simulink model "PNEUMA"  (R2023b)
settings: Solver=ode23tb  StartTime=0  StopTime=3600  FixedStep=0.001  MaxStep=time_step_new  RelTol=0.01  EnableMultiTasking=on
values from neighbouring files (symbols this model uses):
  A = 20.9    [Gas_Exchange_IC.m]    (also in getPneumonia.m = (LF1-LF2)/(1-exp(Rresolve*(t2(end)-t2(1)))))
  a1 = 0.3836    [Dissociation_Spencer_IC.m]    (also in Gas_Exchange_IC.m; Respiratory_IC.m)
  a2 = 1.819    [Dissociation_Spencer_IC.m]    (also in Gas_Exchange_IC.m; Respiratory_IC.m)
  alpha1 = 0.02598    [Dissociation_Spencer_IC.m]    (also in Gas_Exchange_IC.m; Respiratory_IC.m)
  alpha2 = 0.05591    [Dissociation_Spencer_IC.m]    (also in Gas_Exchange_IC.m; Respiratory_IC.m)
  B = 92.8    [Gas_Exchange_IC.m]    (also in getPneumonia.m = LungFunction(end)-A)
  beta1 = 0.012275    [Dissociation_Spencer_IC.m]    (also in Gas_Exchange_IC.m; Respiratory_IC.m)
  beta2 = 0.03255    [Dissociation_Spencer_IC.m]    (also in Gas_Exchange_IC.m; Respiratory_IC.m)
  C = 10570    [Gas_Exchange_IC.m]
  C1 = 9    [Dissociation_Spencer_IC.m]    (also in Gas_Exchange_IC.m; Respiratory_IC.m)
  C2 = 87.00    (= 87)    [Dissociation_Spencer_IC.m]    (also in Gas_Exchange_IC.m; Respiratory_IC.m)
  Circadian_Period = 24    [Respiratory_IC.m]    (also in State_UA_Khoo_IC.m)
  CvCO2IC = 0.5116    [Body_Khoo_IC.m]    (also in Gas_Exchange_IC.m; Respiratory_IC.m = 0.5247)
  CvO2IC = 0.1672    [Body_Khoo_IC.m]    (also in Gas_Exchange_IC.m; Respiratory_IC.m = 0.1639)
  D = -5.251    [Gas_Exchange_IC.m]
  Dead1CO2IC = 0.1020    (= 0.102)    [Dead_Space_Khoo_IC.m]    (also in Gas_Exchange_IC.m; Respiratory_IC.m = 39.5616)
  Dead1O2IC = 149.8824    [Dead_Space_Khoo_IC.m]    (also in Gas_Exchange_IC.m; Respiratory_IC.m = 104.3637)
  Dead2CO2IC = 0.5274    [Dead_Space_Khoo_IC.m]    (also in Gas_Exchange_IC.m; Respiratory_IC.m = 39.6736)
  Dead2O2IC = 149.3923    [Dead_Space_Khoo_IC.m]    (also in Gas_Exchange_IC.m; Respiratory_IC.m = 104.2258)
  Dead3CO2IC = 2.2996    [Dead_Space_Khoo_IC.m]    (also in Gas_Exchange_IC.m; Respiratory_IC.m = 39.8127)
  Dead3O2IC = 147.3503    [Dead_Space_Khoo_IC.m]    (also in Gas_Exchange_IC.m; Respiratory_IC.m = 104.0505)
  Dead4CO2IC = 8.2293    [Dead_Space_Khoo_IC.m]    (also in Gas_Exchange_IC.m; Respiratory_IC.m = 40.0061)
  Dead4O2IC = 140.5179    [Dead_Space_Khoo_IC.m]    (also in Gas_Exchange_IC.m; Respiratory_IC.m = 103.8005)
  Dead5CO2IC = 22.0757    [Dead_Space_Khoo_IC.m]    (also in Gas_Exchange_IC.m; Respiratory_IC.m = 40.3359)
  Dead5O2IC = 124.5641    [Dead_Space_Khoo_IC.m]    (also in Gas_Exchange_IC.m; Respiratory_IC.m = 103.3579)
  DtotalIC = 0.3    [NeuroMuscular_IC.m]    (also in Respiratory_IC.m = 0.32)
  E_CW = 5    [Pleural_Schuessler_IC.m]    (also in Pmus_Flow_Younes_IC.m; Resp_Mech_IC.m; Respiratory_IC.m)
  E_L = 5    [Pleural_Schuessler_IC.m]    (also in Pmus_Flow_Younes_IC.m; Resp_Mech_IC.m; Respiratory_IC.m)
  fc = 0.4/60    (= 0.00666666666667)    [Respiratory_IC.m]    (also in State_UA_Khoo_IC.m)
  fcs_max = 47.78    [Cardiovascular_IC.m]    (also in Reflex_Ursino_IC.m)
  fcs_min = 2.52    [Cardiovascular_IC.m]    (also in Reflex_Ursino_IC.m)
  fcs_zero = 25    [Respiratory_IC.m]
  FlowIC = 0    [Pmus_Flow_Younes_IC.m]    (also in Resp_Mech_IC.m; Respiratory_IC.m)
  fp_inf = 6.3    [Respiratory_IC.m]
  fp_zero = 3.2    [Respiratory_IC.m]
  fs_inf = 2.10    (= 2.1)    [Respiratory_IC.m]
  fs_zero = 16.11    [Respiratory_IC.m]
  ftbs_min = 0.1    [Cardiovascular_IC.m]    (also in SA_Node_Ursino_IC.m)
  gc = 0.008/60    (= 0.000133333333333)    [Respiratory_IC.m]    (also in State_UA_Khoo_IC.m)
  h = 0.0183    [Brain_Khoo_IC.m]    (also in Gas_Exchange_IC.m; Respiratory_IC.m)
  HP_basal = 0.58    [Cardiovascular_IC.m]    (also in SA_Node_Ursino_IC.m)
  Ic = 45    [Gas_Exchange_IC.m]    (also in Respiratory_IC.m; Vent_Drive_Khoo_IC.m)
  IpCO2 = 38    [Gas_Exchange_IC.m]    (also in Respiratory_IC.m; Vent_Drive_Khoo_IC.m)
  IpO2 = 102.4    [Gas_Exchange_IC.m]    (also in Respiratory_IC.m; Vent_Drive_Khoo_IC.m)
  K1 = 13    [Dissociation_Spencer_IC.m]    (also in Gas_Exchange_IC.m; Respiratory_IC.m)
  K2 = 194.4    [Dissociation_Spencer_IC.m]    (also in Gas_Exchange_IC.m; Respiratory_IC.m)
  k_cs = 11.758    [Cardiovascular_IC.m]    (also in Reflex_Ursino_IC.m)
  k_p = 7.06    [Respiratory_IC.m]
  k_s = 0.07    [Respiratory_IC.m]
  lambda = 863    [Gas_Exchange_IC.m]    (also in Lungs_Khoo_IC.m; Respiratory_IC.m)
  Mech_Vent_pressure = 17    [Mech_vent_test.m]
  MRbCO2 = 0.0517    [Brain_Khoo_IC.m]    (also in Gas_Exchange_IC.m; Respiratory_IC.m)
  MRCO2 = 0.0033    [Body_Khoo_IC.m]    (also in Gas_Exchange_IC.m; Respiratory_IC.m)
  MRO2 = 0.0038    [Body_Khoo_IC.m]    (also in Gas_Exchange_IC.m; Respiratory_IC.m)
  NM_block_gain = 1    [Mech_vent_test.m]
  PACO2_delayIC = 39.6041    [Cardio_Mix_Lange_IC.m]    (also in Gas_Exchange_IC.m; Respiratory_IC.m = 40.4448)
  PaCO2firstIC = 0.2150    (= 0.215)    [Cardio_Mix_Lange_IC.m]    (also in Gas_Exchange_IC.m; Respiratory_IC.m = -0.2465)
  PACO2IC = 37.1484    [Gas_Exchange_IC.m]    (also in Lungs_Khoo_IC.m; Respiratory_IC.m = 40.9432)
  PaCO2secondIC = 38.4577    [Cardio_Mix_Lange_IC.m]    (also in Gas_Exchange_IC.m; Respiratory_IC.m = 40.3928)
  PAO2_delayIC = 103.8436    [Cardio_Mix_Lange_IC.m]    (also in Gas_Exchange_IC.m; Respiratory_IC.m = 103.1223)
  PaO2firstIC = -0.2838    [Cardio_Mix_Lange_IC.m]    (also in Gas_Exchange_IC.m; Respiratory_IC.m = 0.3557)
  PAO2IC = 107.1983    [Gas_Exchange_IC.m]    (also in Lungs_Khoo_IC.m; Respiratory_IC.m = 102.5153)
  PaO2secondIC = 105.4828    [Cardio_Mix_Lange_IC.m]    (also in Gas_Exchange_IC.m; Respiratory_IC.m = 103.1435)
  PbCO2IC = 48.2858    [Brain_Khoo_IC.m]    (also in Gas_Exchange_IC.m; Respiratory_IC.m = 48.5383)
  PICO2 = 0    [Dead_Space_Khoo_IC.m]    (also in Gas_Exchange_IC.m; Respiratory_IC.m)
  PIO2 = 150    [Dead_Space_Khoo_IC.m]    (also in Gas_Exchange_IC.m; Respiratory_IC.m)
  PIO2_change = -90    [Mech_vent_test.m]    (also in Respiratory_IC.m = 0)
  Pn = 90    [Cardiovascular_IC.m]    (also in Reflex_Ursino_IC.m)
  Pt_frcIC1 = 0    [Pmus_Flow_Younes_IC.m]    (also in Resp_Mech_IC.m; Respiratory_IC.m)
  Pt_frcIC2 = 0    [Pmus_Flow_Younes_IC.m]    (also in Resp_Mech_IC.m; Respiratory_IC.m)
  QdBo = 0.8333    [Brain_Khoo_IC.m]    (also in Gas_Exchange_IC.m; Respiratory_IC.m)
  R_AW = 1.27    [Pleural_Schuessler_IC.m]    (also in Pmus_Flow_Younes_IC.m; Resp_Mech_IC.m; Respiratory_IC.m)
  R_CW = 1.03    [Pleural_Schuessler_IC.m]    (also in Pmus_Flow_Younes_IC.m; Resp_Mech_IC.m; Respiratory_IC.m)
  R_L = 1.69    [Pleural_Schuessler_IC.m]    (also in Pmus_Flow_Younes_IC.m; Resp_Mech_IC.m; Respiratory_IC.m)
  RC = 0.06    [Pleural_Schuessler_IC.m]    (also in Pmus_Flow_Younes_IC.m; Resp_Mech_IC.m; Respiratory_IC.m)
  rc = 0.2/60    (= 0.00333333333333)    [Respiratory_IC.m]    (also in State_UA_Khoo_IC.m)
  SbCO2 = 0.3600    (= 0.36)    [Brain_Khoo_IC.m]    (also in Gas_Exchange_IC.m; Respiratory_IC.m)
  SCO2 = 0.0043    [Brain_Khoo_IC.m]    (also in Gas_Exchange_IC.m; Respiratory_IC.m)
  SWAo = 0.007    [Respiratory_IC.m]    (also in State_UA_Khoo_IC.m)
  T1 = 1    [Cardio_Mix_Lange_IC.m]    (also in Gas_Exchange_IC.m; Respiratory_IC.m)
  T2 = 2    [Cardio_Mix_Lange_IC.m]    (also in Gas_Exchange_IC.m; Respiratory_IC.m)
  t_end_new = 4*24*60*60    (= 345600)    [Mech_vent_test.m]
  t_end_UA = 0    [Respiratory_IC.m]    (also in State_UA_Khoo_IC.m)
  t_Mech_Vent_duration = 0    [Mech_vent_test.m]
  t_Mech_Vent_start = 0    [Mech_vent_test.m]
  t_Mueller_duration = 0    [NeuroMuscular_IC.m]
  t_Mueller_insp = 0    [NeuroMuscular_IC.m]
  t_Mueller_start = 0    [NeuroMuscular_IC.m]
  t_NM_block_duration = 0    [Mech_vent_test.m]
  t_NM_block_start = 0    [Mech_vent_test.m]
  t_O2_duration = 0    [Mech_vent_test.m]    (also in Respiratory_IC.m)
  t_O2_start = 0    [Mech_vent_test.m]    (also in Respiratory_IC.m)
  t_start_new = 0    [Mech_vent_test.m]
  t_start_UA = 0    [Respiratory_IC.m]    (also in State_UA_Khoo_IC.m)
  t_valsalva_duration = 0    [NeuroMuscular_IC.m]
  t_valsalva_insp = 0    [NeuroMuscular_IC.m]
  t_valsalva_start = 0    [NeuroMuscular_IC.m]
  time_step = time_step    [acquire_data.m]    (also in acquire_data_save.m)
  VC = 5    [Pmus_Flow_Younes_IC.m]    (also in Resp_Mech_IC.m; Respiratory_IC.m)
  Vdead1 = 0.03    [Dead_Space_Khoo_IC.m]    (also in Gas_Exchange_IC.m; Respiratory_IC.m)
  Vdead2 = 0.03    [Dead_Space_Khoo_IC.m]    (also in Gas_Exchange_IC.m; Respiratory_IC.m)
  Vdead3 = 0.03    [Dead_Space_Khoo_IC.m]    (also in Gas_Exchange_IC.m; Respiratory_IC.m)
  Vdead4 = 0.03    [Dead_Space_Khoo_IC.m]    (also in Gas_Exchange_IC.m; Respiratory_IC.m)
  Vdead5 = 0.03    [Dead_Space_Khoo_IC.m]    (also in Gas_Exchange_IC.m; Respiratory_IC.m)
  Ventilator_rate = 12    [Mech_vent_test.m]
  VTCO2 = 15    [Body_Khoo_IC.m]    (also in Gas_Exchange_IC.m; Respiratory_IC.m)
  VtIC = 0    [Pmus_Flow_Younes_IC.m]    (also in Resp_Mech_IC.m; Respiratory_IC.m)
  VTO2 = 6    [Body_Khoo_IC.m]    (also in Gas_Exchange_IC.m; Respiratory_IC.m)
  Z = 0.0227    [Dissociation_Spencer_IC.m]    (also in Gas_Exchange_IC.m; Respiratory_IC.m)
undefined symbols (not defined in the file or in its folder): A_0_ua, alpha_E_FFA_Heart, alpha_E_FFA_muscle, alpha_E_GLC_Heart, alpha_E_GLC_muscle, alpha_E_GLY_muscle, alpha_E_PYR_muscle, alpha_E_TGL_adipose, alpha_E_TGL_GI, alpha_E_TGL_Heart, alpha_E_TGL_muscle, Arousal_UAIC, C_ua_awake, Cbp, Cbv, Ce_0, Cep, Cev, Chp, Chv, Cla, Clamp_class, Cmp, Cmv, Cpa, CPAP_pressure, Cpp, Cpv, Cra, Csa, Csp, Csv, CvbO2_n, CvhO2_n, CvmO2_n, DAY, delay, DietBlock, Dx, Fb, fchemo_max, fchemo_min, fchemoIC, flsIC, Ftas_I0, ftas_min, ftas_r0, FVC_activation, gain_E, Gamma, Gas_sleep, Gas_sleepM, Gb, Gblock, GbO2, Gbs_sleep, gcc_sa, gcc_sb, gcc_sp, Gclamp ... (+144)
libraries: simulink x4, dspstat3 x4, simulink_extras x2
(part 5 of 8)

== system PNEUMA/Display Panels/Saving CARDIORESPIRATORY/If Action Subsystem ==
  In1 : Inport
  Action Port : ActionPort  ActionPortLabel=if((u1>777600)&(u1<=864000))
  "SI/HR/ABP To File " : ToFile  Filename=CARDIORESPIRATORYday10.mat  MatrixName=CARDIORESPIRATORY
  wires:
  In1/1 -> "SI/HR/ABP To File "/1

== system PNEUMA/Display Panels/Saving CARDIORESPIRATORY/Switch Case Action Subsystem ==
  In1 : Inport
  Action Port : ActionPort  ActionPortLabel=case [ 0 ]:
  To File : ToFile  Filename=CARDIORESPIRATORY1.mat  MatrixName=CARDIORESPIRATORY  SampleTime=sampletime
  wires:
  In1/1 -> To File/1

== system PNEUMA/Display Panels/Saving CARDIORESPIRATORY/Switch Case Action Subsystem1 ==
  In1 : Inport
  Action Port : ActionPort  ActionPortLabel=case [ 1 ]:
  To File : ToFile  Filename=CARDIORESPIRATORY2.mat  MatrixName=CARDIORESPIRATORY  SampleTime=sampletime
  wires:
  In1/1 -> To File/1

== system PNEUMA/Display Panels/Saving CARDIORESPIRATORY/Switch Case Action Subsystem2 ==
  In1 : Inport
  Action Port : ActionPort  ActionPortLabel=case [ 2 ]:
  To File : ToFile  Filename=CARDIORESPIRATORY3.mat  MatrixName=CARDIORESPIRATORY  SampleTime=sampletime
  wires:
  In1/1 -> To File/1

== system PNEUMA/Display Panels/Saving CARDIORESPIRATORY/Switch Case Action Subsystem3 ==
  In1 : Inport
  Action Port : ActionPort  ActionPortLabel=default:
  To File : ToFile  Filename=CARDIORESPIRATORY10.mat  MatrixName=CARDIORESPIRATORY  SampleTime=sampletime
  wires:
  In1/1 -> To File/1

== system PNEUMA/Display Panels/Saving CARDIORESPIRATORY/Switch Case Action Subsystem4 ==
  In1 : Inport
  Action Port : ActionPort  ActionPortLabel=case [ 3 ]:
  To File : ToFile  Filename=CARDIORESPIRATORY4.mat  MatrixName=CARDIORESPIRATORY  SampleTime=sampletime
  wires:
  In1/1 -> To File/1

== system PNEUMA/Display Panels/Saving CARDIORESPIRATORY/Switch Case Action Subsystem5 ==
  In1 : Inport
  Action Port : ActionPort  ActionPortLabel=case [ 4 ]:
  To File : ToFile  Filename=CARDIORESPIRATORY5.mat  MatrixName=CARDIORESPIRATORY  SampleTime=sampletime
  wires:
  In1/1 -> To File/1

== system PNEUMA/Display Panels/Saving CARDIORESPIRATORY/Switch Case Action Subsystem6 ==
  In1 : Inport
  Action Port : ActionPort  ActionPortLabel=case [ 5 ]:
  To File : ToFile  Filename=CARDIORESPIRATORY6.mat  MatrixName=CARDIORESPIRATORY  SampleTime=sampletime
  wires:
  In1/1 -> To File/1

== system PNEUMA/Display Panels/Saving CARDIORESPIRATORY/Switch Case Action Subsystem7 ==
  In1 : Inport
  Action Port : ActionPort  ActionPortLabel=case [ 6 ]:
  To File : ToFile  Filename=CARDIORESPIRATORY7.mat  MatrixName=CARDIORESPIRATORY  SampleTime=sampletime
  wires:
  In1/1 -> To File/1

== system PNEUMA/Display Panels/Saving CARDIORESPIRATORY/Switch Case Action Subsystem8 ==
  In1 : Inport
  Action Port : ActionPort  ActionPortLabel=case [ 7 ]:
  To File : ToFile  Filename=CARDIORESPIRATORY8.mat  MatrixName=CARDIORESPIRATORY  SampleTime=sampletime
  wires:
  In1/1 -> To File/1

== system PNEUMA/Display Panels/Saving CARDIORESPIRATORY/Switch Case Action Subsystem9 ==
  In1 : Inport
  Action Port : ActionPort  ActionPortLabel=case [ 8 ]:
  To File : ToFile  Filename=CARDIORESPIRATORY9.mat  MatrixName=CARDIORESPIRATORY  SampleTime=sampletime
  wires:
  In1/1 -> To File/1

== system PNEUMA/Display Panels/Saving CARDIO/Switch Case Action Subsystem ==
  In1 : Inport
  Action Port : ActionPort  ActionPortLabel=case [ 0 ]:
  To File : ToFile  Filename=CARDIO1.mat  MatrixName=CARDIO  SampleTime=sampletime
  wires:
  In1/1 -> To File/1

== system PNEUMA/Display Panels/Saving CARDIO/Switch Case Action Subsystem1 ==
  In1 : Inport
  Action Port : ActionPort  ActionPortLabel=case [ 1 ]:
  To File : ToFile  Filename=CARDIO2.mat  MatrixName=CARDIO  SampleTime=sampletime
  wires:
  In1/1 -> To File/1

== system PNEUMA/Display Panels/Saving CARDIO/Switch Case Action Subsystem2 ==
  In1 : Inport
  Action Port : ActionPort  ActionPortLabel=case [ 2 ]:
  To File : ToFile  Filename=CARDIO3.mat  MatrixName=CARDIO  SampleTime=sampletime
  wires:
  In1/1 -> To File/1

== system PNEUMA/Display Panels/Saving CARDIO/Switch Case Action Subsystem3 ==
  In1 : Inport
  Action Port : ActionPort  ActionPortLabel=default:
  To File : ToFile  Filename=CARDIO10.mat  MatrixName=CARDIO  SampleTime=sampletime
  wires:
  In1/1 -> To File/1

== system PNEUMA/Display Panels/Saving CARDIO/Switch Case Action Subsystem4 ==
  In1 : Inport
  Action Port : ActionPort  ActionPortLabel=case [ 3 ]:
  To File : ToFile  Filename=CARDIO4.mat  MatrixName=CARDIO  SampleTime=sampletime
  wires:
  In1/1 -> To File/1

== system PNEUMA/Display Panels/Saving CARDIO/Switch Case Action Subsystem5 ==
  In1 : Inport
  Action Port : ActionPort  ActionPortLabel=case [ 4 ]:
  To File : ToFile  Filename=CARDIO5.mat  MatrixName=CARDIO  SampleTime=sampletime
  wires:
  In1/1 -> To File/1

== system PNEUMA/Display Panels/Saving CARDIO/Switch Case Action Subsystem6 ==
  In1 : Inport
  Action Port : ActionPort  ActionPortLabel=case [ 5 ]:
  To File : ToFile  Filename=CARDIO6.mat  MatrixName=CARDIO  SampleTime=sampletime
  wires:
  In1/1 -> To File/1

== system PNEUMA/Display Panels/Saving CARDIO/Switch Case Action Subsystem7 ==
  In1 : Inport
  Action Port : ActionPort  ActionPortLabel=case [ 6 ]:
  To File : ToFile  Filename=CARDIO7.mat  MatrixName=CARDIO  SampleTime=sampletime
  wires:
  In1/1 -> To File/1

== system PNEUMA/Display Panels/Saving CARDIO/Switch Case Action Subsystem8 ==
  In1 : Inport
  Action Port : ActionPort  ActionPortLabel=case [ 7 ]:
  To File : ToFile  Filename=CARDIO8.mat  MatrixName=CARDIO  SampleTime=sampletime
  wires:
  In1/1 -> To File/1

== system PNEUMA/Display Panels/Saving CARDIO/Switch Case Action Subsystem9 ==
  In1 : Inport
  Action Port : ActionPort  ActionPortLabel=case [ 8 ]:
  To File : ToFile  Filename=CARDIO9.mat  MatrixName=CARDIO  SampleTime=sampletime
  wires:
  In1/1 -> To File/1

== system PNEUMA/Metabolic Control/Display & Storage/Saving G_I_FFA ==
  In1 : Inport
  Clock : Clock
  Gain = 7day : Gain  Gain=1/(3600*24*DAY)
  Rounding Function : Rounding
  Switch Case : SwitchCase  CaseConditions={0,1,2,3,4,5,6,7,8}  SampleTime=sampletime*6
  Switch Case Action Subsystem : Subsystem  TreatAsAtomicUnit=on
  Switch Case Action Subsystem1 : Subsystem  TreatAsAtomicUnit=on
  Switch Case Action Subsystem2 : Subsystem  TreatAsAtomicUnit=on
  Switch Case Action Subsystem3 : Subsystem  TreatAsAtomicUnit=on
  Switch Case Action Subsystem4 : Subsystem  TreatAsAtomicUnit=on
  Switch Case Action Subsystem5 : Subsystem  TreatAsAtomicUnit=on
  Switch Case Action Subsystem6 : Subsystem  TreatAsAtomicUnit=on
  Switch Case Action Subsystem7 : Subsystem  TreatAsAtomicUnit=on
  Switch Case Action Subsystem8 : Subsystem  TreatAsAtomicUnit=on
  Switch Case Action Subsystem9 : Subsystem  TreatAsAtomicUnit=on
  wires:
  Clock/1 -> Gain = 7day/1
  Switch Case/1 -> Switch Case Action Subsystem/Action
  Switch Case/2 -> Switch Case Action Subsystem1/Action
  Switch Case/3 -> Switch Case Action Subsystem2/Action
  Switch Case/10 -> Switch Case Action Subsystem3/Action
  Rounding Function/1 -> Switch Case/1
  In1/1 -> Switch Case Action Subsystem/1(In1), Switch Case Action Subsystem1/1(In1), Switch Case Action Subsystem2/1(In1), Switch Case Action Subsystem4/1(In1), Switch Case Action Subsystem5/1(In1), Switch Case Action Subsystem3/1(In1), Switch Case Action Subsystem9/1(In1), Switch Case Action Subsystem8/1(In1), Switch Case Action Subsystem7/1(In1), Switch Case Action Subsystem6/1(In1)
  Gain = 7day/1 -> Rounding Function/1
  Switch Case/4 -> Switch Case Action Subsystem4/Action
  Switch Case/5 -> Switch Case Action Subsystem5/Action
  Switch Case/6 -> Switch Case Action Subsystem6/Action
  Switch Case/7 -> Switch Case Action Subsystem7/Action
  Switch Case/8 -> Switch Case Action Subsystem8/Action
  Switch Case/9 -> Switch Case Action Subsystem9/Action

== system PNEUMA/Metabolic Control/Epinephrine Regulation on Heart and Muscle/Epi Dynamics ==
  Ftas_r : Inport
  SI : Inport  Port=2
  REM : Inport  Port=3
  Constant1 : Constant  Value=Ce_0
  Ftas_Ce0 : Fcn  Expr=(u(1) - ftas_r0*(1-u(2)*Gas_sleepM)+1)*1e-6
  Ftas_Ce0*(1-SI) : Fcn  Expr=((u(1)>=u(4))*(u(1)-u(4)+0) + (u(1)<u(4))*0)*(1-u(2))*1e-6
  Ftas_Ce0*(1-SI*Gas_SleepM) : Fcn  Expr=((u(1)>=u(4))*(u(1)-u(4)+1) + (u(1)<u(4))*1)*(1-u(2)*Gas_sleepM)*1e-6
  Ftas_REM_Sleeo ABS Fcn REM factor = 0.4 Ftas,r0_metabolic Gas factor_M : Fcn  Expr=(abs(u(1) - ftas_r0*(1-u(2)*Gas_sleepM)+1))^(u(2)*Gas_sleepM)*(1+0.4*u(3))*(1-u(2)*0.6)
  Ftas_REM_Sleep Fcn REM factor = 0.4 Ftas,r0_metabolic Gas factor_M Neg Power : Fcn  Expr=((u(1)>=u(4))*(u(1)-u(4)+1) + (u(1)<u(4))*1)^(-u(2)*Gas_sleepM)*(1+0.4*u(3))*(1-u(2)*0.6)
  Ftas_metabolic : Fcn  Expr=u(1)*(1-u(2)*Gas_sleepM)
  Ftas_r0_metabolic : Fcn  Expr=ftas_r0*(1-u(2)*Gas_sleepM)
  Gain : Gain  Gain=1/tao_e
  Gain1 : Gain  Gain=9
  Integrator : Integrator  InitialCondition=Ce_0
  Mux : Mux  Inputs=2
  Mux1 : Mux
  Product : Product  RndMeth=Zero
  Saturation : Saturate  UpperLimit=3  LowerLimit=0.1
  Sum1 : Sum  Inputs=-++  InputSameDT=on  SaturateOnIntegerOverflow=on  OutDataTypeStr=Inherit: Same as first input
  Terminator : Terminator
  Terminator1 : Terminator
  Terminator2 : Terminator
  Ce(t) : Outport
  W_alphaSYMP : Outport  Port=2
  wires:
  Sum1/1 -> Gain/1
  Integrator/1 -> Sum1/1, Ce(t)/1
  Gain/1 -> Integrator/1
  Constant1/1 -> Product/2
  Product/1 -> Sum1/2
  Mux/1 -> Ftas_r0_metabolic/1, Ftas_metabolic/1
  Ftas_r/1 -> Mux/1
  SI/1 -> Mux/2, Mux1/2
  Ftas_metabolic/1 -> Mux1/1
  REM/1 -> Mux1/3
  Mux1/1 -> Ftas_REM_Sleep Fcn REM factor = 0.4 Ftas,r0_metabolic Gas factor_M Neg Power/1, Ftas_REM_Sleeo ABS Fcn REM factor = 0.4 Ftas,r0_metabolic Gas factor_M/1, Ftas_Ce0*(1-SI)/1, Ftas_Ce0*(1-SI*Gas_SleepM)/1, Ftas_Ce0/1
  Ftas_Ce0/1 -> Terminator1/1
  Ftas_r0_metabolic/1 -> Mux1/4
  Ftas_REM_Sleeo ABS Fcn REM factor = 0.4 Ftas,r0_metabolic Gas factor_M/1 -> Terminator/1
  Ftas_REM_Sleep Fcn REM factor = 0.4 Ftas,r0_metabolic Gas factor_M Neg Power/1 -> Saturation/1
  Saturation/1 -> Product/1, W_alphaSYMP/1
  Gain1/1 -> Sum1/3
  Ftas_Ce0*(1-SI*Gas_SleepM)/1 -> Terminator2/1
  Ftas_Ce0*(1-SI)/1 -> Gain1/1

== system PNEUMA/Metabolic Control/Epinephrine Regulation on Heart and Muscle/Epi Modulation ==
  Ce(t) : Inport
  GI : Subsystem
  GI1 : Subsystem
  Heart : Subsystem
  Heart Fluxes : Scope
  Muscle : Subsystem
  Muscle Fluxes : Scope
  Epi on Heart : Outport
  Epi on Muscle : Outport  Port=2
  Epi on GI : Outport  Port=3
  Epi on adipose : Outport  Port=4
  4Fluxes of Epi in Heart : Outport  Port=5
  5Fluxes of Epi in Muscle : Outport  Port=6
  wires:
  Heart/2(Epi on Heart (Sum)) -> Epi on Heart/1
  Ce(t)/1 -> Heart/1(Ce(t)), Muscle/1(Ce(t)), GI/1(Ce(t)), GI1/1(Ce(t))
  Heart/1(Epi on Heart (Fluxes)) -> Heart Fluxes/1, 4Fluxes of Epi in Heart/1
  Muscle/2(Epi on Muscle(Sum)) -> Epi on Muscle/1
  Muscle/1(Epi on Muscle (Fluxes)) -> Muscle Fluxes/1, 5Fluxes of Epi in Muscle/1
  GI/1(Epi on GI) -> Epi on GI/1
  GI1/1(Epi on adipose) -> Epi on adipose/1

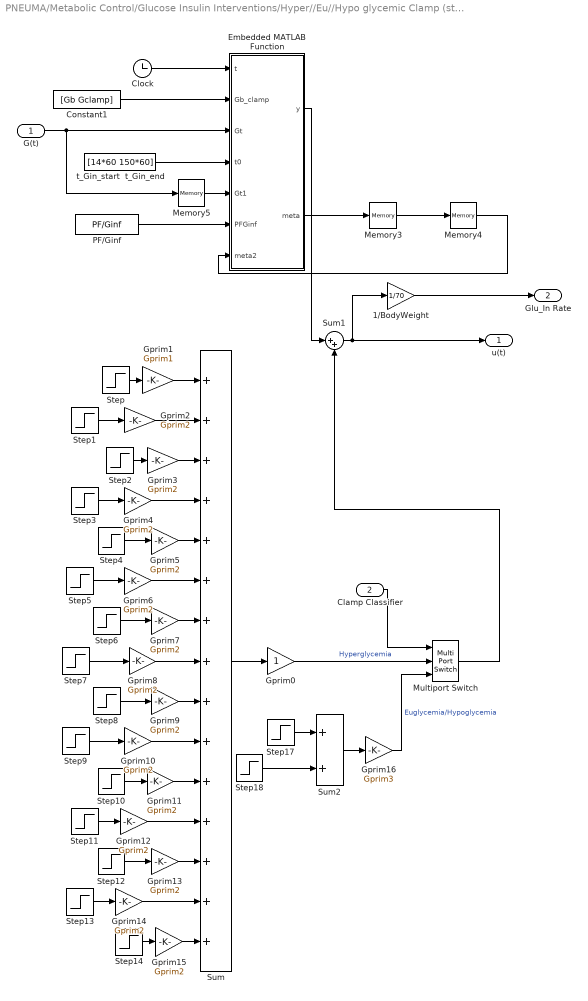
== system PNEUMA/Metabolic Control/Glucose Insulin Interventions/Hyper//Eu//Hypo glycemic Clamp (step by step) ==
  G(t) : Inport
  Clamp Classifier : Inport  Port=2
  1/BodyWeight : Gain  Gain=1/70
  Clock : Clock
  Constant1 : Constant  Value=[Gb Gclamp]
  Embedded MATLAB Function : MATLAB Function  TreatAsAtomicUnit=on
  Gprim0 : Gain
  Gprim1 : Gain  Gain=Gprim1
  Gprim{2..15} (14 alike) : Gain  Gain=Gprim2
  Gprim16 : Gain  Gain=Gprim3
  Memory3 : Memory  InitialCondition=4*70/60
  Memory4 : Memory  InitialCondition=4*70/60
  Memory5 : Memory  InitialCondition=Gb
  Multiport Switch : MultiPortSwitch  Inputs=2  SaturateOnIntegerOverflow=off  InputSameDT=off
  PF/Ginf : Constant  Value=PF/Ginf
  Step : Step  Time=0  After=1768*SurfaceArea  SampleTime=0
  Step1 : Step  Time=1*60  After=(1428-1768)*SurfaceArea  SampleTime=0
  Step10 : Step  Time=10*60  After=(340-374)*SurfaceArea  SampleTime=0
  Step11 : Step  Time=11*60  After=(306-340)*SurfaceArea  SampleTime=0
  Step12 : Step  Time=12*60  After=(272-306)*SurfaceArea  SampleTime=0
  Step13 : Step  Time=13*60  After=(238-272)*SurfaceArea  SampleTime=0
  Step14 : Step  Time=14*60  After=(-238)*SurfaceArea  SampleTime=0
  Step17 : Step  Time=2*60  After=2*70  SampleTime=0
  Step18 : Step  Time=10*60  After=(2.5-2)*70  SampleTime=0
  Step2 : Step  Time=2*60  After=(1156-1428)*SurfaceArea  SampleTime=0
  Step3 : Step  Time=3*60  After=(918-1156)*SurfaceArea  SampleTime=0
  Step4 : Step  Time=4*60  After=(782-918)*SurfaceArea  SampleTime=0
  Step5 : Step  Time=5*60  After=(646-782)*SurfaceArea  SampleTime=0
  Step6 : Step  Time=6*60  After=(544-646)*SurfaceArea  SampleTime=0
  Step7 : Step  Time=7*60  After=(442-544)*SurfaceArea  SampleTime=0
  Step8 : Step  Time=8*60  After=(408-442)*SurfaceArea  SampleTime=0
  Step9 : Step  Time=9*60  After=(374-408)*SurfaceArea  SampleTime=0
  Sum : Sum  Inputs=+++++++++++++++
  Sum1 : Sum  Inputs=|++
  Sum2 : Sum
  t_Gin_start  t_Gin_end : Constant  Value=[14*60 150*60]
  u(t) : Outport
  Glu_In Rate : Outport  Port=2
  wires:
  Clock/1 -> Embedded MATLAB Function/1(t)
  Constant1/1 -> Embedded MATLAB Function/2(Gb_clamp)
  t_Gin_start  t_Gin_end/1 -> Embedded MATLAB Function/4(t0)
  Embedded MATLAB Function/2(meta) -> Memory3/1
  Memory3/1 -> Memory4/1
  Memory5/1 -> Embedded MATLAB Function/5(Gt1)
  Memory4/1 -> Embedded MATLAB Function/7(meta2)
  G(t)/1 -> Embedded MATLAB Function/3(Gt), Memory5/1
  Embedded MATLAB Function/1(y) -> Sum1/1
  1/BodyWeight/1 -> Glu_In Rate/1
  Step/1 -> Gprim1/1
  Step1/1 -> Gprim2/1
  Step2/1 -> Gprim3/1
  Step3/1 -> Gprim4/1
  Step4/1 -> Gprim5/1
  Step5/1 -> Gprim6/1
  Step6/1 -> Gprim7/1
  Step7/1 -> Gprim8/1
  Step8/1 -> Gprim9/1
  Step9/1 -> Gprim10/1
  Step10/1 -> Gprim11/1
  Step11/1 -> Gprim12/1
  Step12/1 -> Gprim13/1
  Step13/1 -> Gprim14/1
  Step14/1 -> Gprim15/1
  Sum/1 -> Gprim0/1
  Sum1/1 -> 1/BodyWeight/1, u(t)/1
  Gprim0/1 -> Multiport Switch/2  "Hyperglycemia"
  Gprim1/1 -> Sum/1
  Gprim2/1 -> Sum/2
  Gprim3/1 -> Sum/3
  Gprim4/1 -> Sum/4
  Gprim5/1 -> Sum/5
  Gprim6/1 -> Sum/6
  Gprim7/1 -> Sum/7
  Gprim8/1 -> Sum/8
  Gprim9/1 -> Sum/9
  Gprim10/1 -> Sum/10
  Gprim11/1 -> Sum/11
  Gprim12/1 -> Sum/12
  Gprim13/1 -> Sum/13
  Gprim14/1 -> Sum/14
  Gprim15/1 -> Sum/15
  Step17/1 -> Sum2/1
  Step18/1 -> Sum2/2
  Sum2/1 -> Gprim16/1
  Clamp Classifier/1 -> Multiport Switch/1
  Multiport Switch/1 -> Sum1/2
  Gprim16/1 -> Multiport Switch/3  "Euglycemia/Hypoglycemia"
  PF/Ginf/1 -> Embedded MATLAB Function/6(PFGinf)

== system PNEUMA/Metabolic Control/Glucose Insulin Interventions/IVGTT ==
  Step : Step  Time=begin_time  After=init_value  SampleTime=0
  Step1 : Step  Time=end_time  After=end_value - init_value  SampleTime=0
  Sum : Sum  Inputs=|++
  Out1 : Outport
  wires:
  Step/1 -> Sum/1
  Step1/1 -> Sum/2
  Sum/1 -> Out1/1

== system PNEUMA/Metabolic Control/Glucose Insulin Interventions/Insulin Pump Euglycemic Clamp ==
  Gprim{1..11} (11 alike) : Gain
  Step : Step  Time=0  After=127.6*SurfaceArea  SampleTime=0
  Step1 : Step  Time=1*60  After=(113.6-127.6)*SurfaceArea  SampleTime=0
  Step10 : Step  Time=10*60  After=(40-45)*SurfaceArea  SampleTime=0
  Step2 : Step  Time=2*60  After=(101.2-113.6)*SurfaceArea  SampleTime=0
  Step3 : Step  Time=3*60  After=(90.2-101.2)*SurfaceArea  SampleTime=0
  Step4 : Step  Time=4*60  After=(80.2-90.2)*SurfaceArea  SampleTime=0
  Step5 : Step  Time=5*60  After=(71.4-80.2)*SurfaceArea  SampleTime=0
  Step6 : Step  Time=6*60  After=(63.6-71.4)*SurfaceArea  SampleTime=0
  Step7 : Step  Time=7*60  After=(56.8-63.4)*SurfaceArea  SampleTime=0
  Step8 : Step  Time=8*60  After=(50.4-56.8)*SurfaceArea  SampleTime=0
  Step9 : Step  Time=9*60  After=(45-50.4)*SurfaceArea  SampleTime=0
  Sum : Sum  Inputs=+++++++++++
  mU to microU : Gain  Gain=In_gain
  Out1 : Outport
  wires:
  Step/1 -> Gprim1/1
  Step1/1 -> Gprim2/1
  Step2/1 -> Gprim3/1
  Step3/1 -> Gprim4/1
  Step4/1 -> Gprim5/1
  Step5/1 -> Gprim6/1
  Step6/1 -> Gprim7/1
  Step7/1 -> Gprim8/1
  Step8/1 -> Gprim9/1
  Step9/1 -> Gprim10/1
  Step10/1 -> Gprim11/1
  Sum/1 -> mU to microU/1
  Gprim1/1 -> Sum/1
  Gprim2/1 -> Sum/2
  Gprim3/1 -> Sum/3
  Gprim4/1 -> Sum/4
  Gprim5/1 -> Sum/5
  Gprim6/1 -> Sum/6
  Gprim7/1 -> Sum/7
  Gprim8/1 -> Sum/8
  Gprim9/1 -> Sum/9
  Gprim10/1 -> Sum/10
  Gprim11/1 -> Sum/11
  mU to microU/1 -> Out1/1

== system PNEUMA/Metabolic Control/Glucose-Insulin-FFA Minimal Model/FFA Dynamics_LC ==
  note: Orinally Design
      | Yb=0.01*Xb
  G(t) : Inport
  Y(t) : Inport  Port=2
  u3(t) : Inport  Port=3
  1/VolF : Gain  Gain=1/VolF  SaturateOnIntegerOverflow=on  OutDataTypeStr=Inherit: Same as input  ParamDataTypeStr=Inherit: Same as input
  Gb*Fb : Gain  Gain=Gb*Fb  SaturateOnIntegerOverflow=on  OutDataTypeStr=Inherit: Same as input  ParamDataTypeStr=Inherit: Same as input
  Int5 : Integrator  InitialCondition=Fb
  Product8 : Product  Inputs=3  InputSameDT=on  RndMeth=Zero  SaturateOnIntegerOverflow=on  OutDataTypeStr=Inherit: Same as first input
  Product9 : Product  Inputs=3  InputSameDT=on  RndMeth=Zero  SaturateOnIntegerOverflow=on  OutDataTypeStr=Inherit: Same as first input
  Sum6 : Sum  Inputs=--++-++  InputSameDT=on  SaturateOnIntegerOverflow=on  OutDataTypeStr=Inherit: Same as first input
  p7 : Gain  Gain=p7  SaturateOnIntegerOverflow=on  OutDataTypeStr=Inherit: Same as input  ParamDataTypeStr=Inherit: Same as input
  p7*Fb : Constant  Value=p7*Fb
  p7*Fb1 : Constant  Value=p8*0.1*Xb*Fb
  p8 : Constant  Value=p8
  p9 : Fcn  Expr=0.00021/60*exp(-0.0055*u)
  F(t) : Outport
  wires:
  Int5/1 -> p7/1, Product8/3, F(t)/1, Product9/3  "F(t)"
  Sum6/1 -> Int5/1
  p8/1 -> Product8/2
  Product8/1 -> Sum6/2
  p9/1 -> Gb*Fb/1, Product9/1
  Product9/1 -> Sum6/3
  p7*Fb/1 -> Sum6/4
  Gb*Fb/1 -> Sum6/5
  1/VolF/1 -> Sum6/6
  p7/1 -> Sum6/1
  G(t)/1 -> p9/1, Product9/2
  u3(t)/1 -> 1/VolF/1
  Y(t)/1 -> Product8/1
  p7*Fb1/1 -> Sum6/7

== system PNEUMA/Metabolic Control/Glucose-Insulin-FFA Minimal Model/Glucose Dynamics_LC ==
  u2(t) : Inport
  Z(t) : Inport  Port=2
  X(t) : Inport  Port=3
  1/VolG : Gain  Gain=1/VolG  SaturateOnIntegerOverflow=on  OutDataTypeStr=Inherit: Same as input  ParamDataTypeStr=Inherit: Same as input
  Integrator : Integrator  InitialCondition=Gb
  Prod : Product  Inputs=3  InputSameDT=on  RndMeth=Zero  SaturateOnIntegerOverflow=on  OutDataTypeStr=Inherit: Same as first input
  Prod1 : Product  Inputs=3  InputSameDT=on  RndMeth=Zero  SaturateOnIntegerOverflow=on  OutDataTypeStr=Inherit: Same as first input
  Sum : Sum  Inputs=-+-+-+  InputSameDT=on  SaturateOnIntegerOverflow=on  OutDataTypeStr=Inherit: Same as first input
  Sum1 : Sum  Inputs=|-+
  p1 : Gain  Gain=p1  SaturateOnIntegerOverflow=on  OutDataTypeStr=Inherit: Same as input  ParamDataTypeStr=Inherit: Same as input
  p1Gb : Constant  Value=Gb
  p4 : Constant  Value=p4
  p6 : Constant  Value=p6
  p6*Gb*Zb : Constant  Value=p6*Gb*Zb
  p6*Gb*Zb1 : Constant  Value=p4*Xb*Gb
  G(t) : Outport
  wires:
  p1/1 -> Sum/1
  Integrator/1 -> Prod/1, Prod1/1, Sum1/2, G(t)/1  "G(t)"
  Sum/1 -> Integrator/1
  p4/1 -> Prod/2
  p6*Gb*Zb/1 -> Sum/3
  p6/1 -> Prod1/2
  Z(t)/1 -> Prod1/3
  p1Gb/1 -> Sum1/1
  Sum1/1 -> p1/1
  Prod/1 -> Sum/5
  Prod1/1 -> Sum/4
  1/VolG/1 -> Sum/2
  u2(t)/1 -> 1/VolG/1
  X(t)/1 -> Prod/3
  p6*Gb*Zb1/1 -> Sum/6

== system PNEUMA/Metabolic Control/Glucose-Insulin-FFA Minimal Model/Insulin Dynamics _ B&P ==
  G(t) : Inport
  u1(t) : Inport  Port=2
  Constant : Constant
  Constant1 : Constant  Value=Ib
  Gamma : Gain  Gain=Gamma  SaturateOnIntegerOverflow=on  OutDataTypeStr=Inherit: Same as input  ParamDataTypeStr=Inherit: Same as input
  "Insulin Destruction Gain, Nu = 0.36" : Gain  Gain=n  SaturateOnIntegerOverflow=on  OutDataTypeStr=Inherit: Same as input  ParamDataTypeStr=Inherit: Same as input
  Int1 : Integrator  InitialCondition=Ib
  Int2 : Integrator  InitialCondition=0.0 - delay
  Product : Product  InputSameDT=on  RndMeth=Zero  SaturateOnIntegerOverflow=on  OutDataTypeStr=Inherit: Same as first input
  Random Number : RandomNumber  Mean=5  Variance=9  Seed=5  SampleTime=0
  Step : Step  Time=0  After=125  SampleTime=0
  Step1 : Step  Time=8*60  After=Gh-125  SampleTime=0
  Sum1 : Sum  Inputs=+-  InputSameDT=on  SaturateOnIntegerOverflow=on  OutDataTypeStr=Inherit: Same as first input
  Sum14 : Sum  Inputs=|++
  Sum2 : Sum  Inputs=+-  InputSameDT=on  SaturateOnIntegerOverflow=on  OutDataTypeStr=Inherit: Same as first input
  Sum3 : Sum  Inputs=++-  InputSameDT=on  SaturateOnIntegerOverflow=on  OutDataTypeStr=Inherit: Same as first input
  Terminator1 : Terminator
  Threshold Glucose Concentration (h) : Constant  Value=Gb
  Thresholding Operator1 : Saturate  UpperLimit=100000  LowerLimit=0
  Thresholding Operator2 : Saturate  UpperLimit=20/60  LowerLimit=0
  Variable Time Delay : VariableTransportDelay  VariableDelayType=Variable transport delay  MaximumDelay=10  MaximumPoints=1024*5
  p5 : Gain  Gain=p5  SaturateOnIntegerOverflow=on  OutDataTypeStr=Inherit: Same as input  ParamDataTypeStr=Inherit: Same as input
  I(t) : Outport
  wires:
  Int1/1 -> I(t)/1, Sum1/1
  Sum3/1 -> Int1/1
  "Insulin Destruction Gain, Nu = 0.36"/1 -> Sum3/3
  Gamma/1 -> Thresholding Operator1/1
  Sum2/1 -> Gamma/1
  Constant/1 -> Int2/1
  Product/1 -> Thresholding Operator2/1
  Int2/1 -> Product/2
  G(t)/1 -> Sum2/1
  u1(t)/1 -> p5/1
  p5/1 -> Sum3/2
  Sum1/1 -> "Insulin Destruction Gain, Nu = 0.36"/1
  Constant1/1 -> Sum1/2
  Thresholding Operator2/1 -> Sum3/1
  Thresholding Operator1/1 -> Variable Time Delay/1
  Variable Time Delay/1 -> Product/1
  Random Number/1 -> Variable Time Delay/2
  Step/1 -> Sum14/1
  Step1/1 -> Sum14/2
  Sum14/1 -> Sum2/2
  Threshold Glucose Concentration (h)/1 -> Terminator1/1

== system PNEUMA/Metabolic Control/Glucose-Insulin-FFA Minimal Model/Remote Compartment p3 // (s + p2)1 ==
  I(t) : Inport
  Int4 : Integrator  InitialCondition=Xb
  Sum5 : Sum  Inputs=-+-+  InputSameDT=on  SaturateOnIntegerOverflow=on  OutDataTypeStr=Inherit: Same as first input
  k1*Fb : Constant  Value=p3*Ib
  k2 : Gain  Gain=p2  SaturateOnIntegerOverflow=on  OutDataTypeStr=Inherit: Same as input  ParamDataTypeStr=Inherit: Same as input
  k2*Zb : Constant  Value=p2*Xb
  p3 : Gain  Gain=p3  SaturateOnIntegerOverflow=on  OutDataTypeStr=Inherit: Same as input  ParamDataTypeStr=Inherit: Same as input
  X(t) : Outport
  wires:
  Sum5/1 -> Int4/1
  k1*Fb/1 -> Sum5/1
  k2*Zb/1 -> Sum5/2
  k2/1 -> Sum5/3
  Int4/1 -> k2/1, X(t)/1
  p3/1 -> Sum5/4
  I(t)/1 -> p3/1

== system PNEUMA/Metabolic Control/Glucose-Insulin-FFA Minimal Model/Remote Ins_FFA pF3 // (s + pF2) ==
  note: Orinally Design
      | Yb=0.01*Xb
  I(t) : Inport
  Int4 : Integrator  InitialCondition=Xb*0.8
  Sum5 : Sum  Inputs=-+-+  InputSameDT=on  SaturateOnIntegerOverflow=on  OutDataTypeStr=Inherit: Same as first input
  k1*Fb : Constant  Value=pF3*Ib
  k2 : Gain  Gain=pF2  SaturateOnIntegerOverflow=on  OutDataTypeStr=Inherit: Same as input  ParamDataTypeStr=Inherit: Same as input
  k2*Zb : Constant  Value=pF2*Xb*0.1
  p3 : Gain  Gain=pF3  SaturateOnIntegerOverflow=on  OutDataTypeStr=Inherit: Same as input  ParamDataTypeStr=Inherit: Same as input
  Y(t) : Outport
  wires:
  Sum5/1 -> Int4/1
  k1*Fb/1 -> Sum5/1
  k2*Zb/1 -> Sum5/2
  k2/1 -> Sum5/3
  Int4/1 -> k2/1, Y(t)/1
  p3/1 -> Sum5/4
  I(t)/1 -> p3/1

== system PNEUMA/Metabolic Control/Glucose-Insulin-FFA Minimal Model/Saving deltaFtas_WalphaSYMP ==
  In1 : Inport
  Clock : Clock
  Gain : Gain  Gain=1/(3600*24*DAY)
  Rounding Function : Rounding
  Switch Case : SwitchCase  CaseConditions={0,1,2,3,4,5,6,7,8}  SampleTime=sampletime
  Switch Case Action Subsystem : Subsystem  TreatAsAtomicUnit=on
  Switch Case Action Subsystem1 : Subsystem  TreatAsAtomicUnit=on
  Switch Case Action Subsystem2 : Subsystem  TreatAsAtomicUnit=on
  Switch Case Action Subsystem3 : Subsystem  TreatAsAtomicUnit=on
  Switch Case Action Subsystem4 : Subsystem  TreatAsAtomicUnit=on
  Switch Case Action Subsystem5 : Subsystem  TreatAsAtomicUnit=on
  Switch Case Action Subsystem6 : Subsystem  TreatAsAtomicUnit=on
  Switch Case Action Subsystem7 : Subsystem  TreatAsAtomicUnit=on
  Switch Case Action Subsystem8 : Subsystem  TreatAsAtomicUnit=on
  Switch Case Action Subsystem9 : Subsystem  TreatAsAtomicUnit=on
  wires:
  Clock/1 -> Gain/1
  Switch Case/1 -> Switch Case Action Subsystem/Action
  Switch Case/2 -> Switch Case Action Subsystem1/Action
  Switch Case/3 -> Switch Case Action Subsystem2/Action
  Switch Case/10 -> Switch Case Action Subsystem3/Action
  Rounding Function/1 -> Switch Case/1
  In1/1 -> Switch Case Action Subsystem/1(In1), Switch Case Action Subsystem1/1(In1), Switch Case Action Subsystem2/1(In1), Switch Case Action Subsystem5/1(In1), Switch Case Action Subsystem3/1(In1), Switch Case Action Subsystem9/1(In1), Switch Case Action Subsystem8/1(In1), Switch Case Action Subsystem7/1(In1), Switch Case Action Subsystem6/1(In1), Switch Case Action Subsystem4/1(In1)
  Gain/1 -> Rounding Function/1
  Switch Case/4 -> Switch Case Action Subsystem4/Action
  Switch Case/5 -> Switch Case Action Subsystem5/Action
  Switch Case/6 -> Switch Case Action Subsystem6/Action
  Switch Case/7 -> Switch Case Action Subsystem7/Action
  Switch Case/8 -> Switch Case Action Subsystem8/Action
  Switch Case/9 -> Switch Case Action Subsystem9/Action

== system PNEUMA/Metabolic Control/Glucose-Insulin-FFA Minimal Model/Subsystem ==
  F(t) : Inport
  Int4 : Integrator  InitialCondition=Zb
  Sum5 : Sum  Inputs=-+-+  InputSameDT=on  SaturateOnIntegerOverflow=on  OutDataTypeStr=Inherit: Same as first input
  k1 : Gain  Gain=k1  SaturateOnIntegerOverflow=on  OutDataTypeStr=Inherit: Same as input  ParamDataTypeStr=Inherit: Same as input
  k1*Fb : Constant  Value=k1*Fb
  k2 : Gain  Gain=k2  SaturateOnIntegerOverflow=on  OutDataTypeStr=Inherit: Same as input  ParamDataTypeStr=Inherit: Same as input
  k2*Zb : Constant  Value=k2*Zb
  Z(t) : Outport
  wires:
  Sum5/1 -> Int4/1
  k1*Fb/1 -> Sum5/1
  k2*Zb/1 -> Sum5/2
  k2/1 -> Sum5/3
  Int4/1 -> k2/1, Z(t)/1
  k1/1 -> Sum5/4
  F(t)/1 -> k1/1

== system PNEUMA/Respiratory System/Gas Exchange/BODY TISSUES COMPARTMENT ==
  SI Sleep Wake State Index : Inport
  CaCO2 : Inport  Port=2
  CaO2 : Inport  Port=3
  "Qt " : Inport  Port=4
  Body Tissues Compartment for CO2 : Subsystem
  Body Tissues Compartment for O2 : Subsystem
  CvCO2 : Outport
  CvO2 : Outport  Port=2
  wires:
  SI Sleep Wake State Index/1 -> Body Tissues Compartment for CO2/3(SI Sleep Wake State Index), Body Tissues Compartment for O2/2(SI Sleep Wake State Index)
  CaCO2/1 -> Body Tissues Compartment for CO2/1(CaCO2)
  CaO2/1 -> Body Tissues Compartment for O2/3(CaO2)
  Body Tissues Compartment for CO2/1(CvCO2) -> CvCO2/1
  Body Tissues Compartment for O2/1(CVO2) -> CvO2/1
  "Qt "/1 -> Body Tissues Compartment for O2/1(Qt), Body Tissues Compartment for CO2/2(Qt)

== system PNEUMA/Respiratory System/Gas Exchange/BRAIN COMPARTMENT ==
  Qb : Inport
  PaCO2 : Inport  Port=2
  SI Sleep Wake State Index : Inport  Port=3
  Fcn : Fcn  Expr=MRbCO2*(0.375*(1-0.4*u)+0.625)
  Fcn -5 blocks : Fcn  Expr=(u(1) + ( u(2) * u(3)) *SCO2- h ) /SbCO2
  Integrator : Integrator  InitialCondition=PbCO2IC
  Mux : Mux  Inputs=3
  sum : Sum  Inputs=+-  InputSameDT=on  SaturateOnIntegerOverflow=on  OutDataTypeStr=Inherit: Same as first input
  PbCO2 : Outport
  tag scope: PbCO2IC=global
  wires:
  Fcn -5 blocks/1 -> Integrator/1
  PaCO2/1 -> sum/1
  Integrator/1 -> sum/2, [PbCO2IC], PbCO2/1
  SI Sleep Wake State Index/1 -> Fcn/1
  Mux/1 -> Fcn -5 blocks/1
  Fcn/1 -> Mux/1
  Qb/1 -> Mux/2
  sum/1 -> Mux/3

== system PNEUMA/Respiratory System/Gas Exchange/Cardiovascular Mixing and Convection ==
  Lung-Chemoreceptor Delay Volume : Inport
  PACO2 : Inport  Port=2
  PAO2 : Inport  Port=3
  Q : Inport  Port=4
  CO2 Cardiovascular Mixing and Convection Effects : Subsystem
  O2 Cardiovascular Mixing and Convection Effects : Subsystem
  PaCO2 : Outport
  PaO2 : Outport  Port=2
  wires:
  CO2 Cardiovascular Mixing and Convection Effects/1(PaCO2) -> PaCO2/1
  PACO2/1 -> CO2 Cardiovascular Mixing and Convection Effects/1(PACO2)
  Q/1 -> CO2 Cardiovascular Mixing and Convection Effects/2(Q), O2 Cardiovascular Mixing and Convection Effects/1(Q)
  Lung-Chemoreceptor Delay Volume/1 -> CO2 Cardiovascular Mixing and Convection Effects/3(Lung-Chemoreceptor Delay Volume), O2 Cardiovascular Mixing and Convection Effects/3(Lung-Chemoreceptor Delay Volume)
  O2 Cardiovascular Mixing and Convection Effects/1(PaO2) -> PaO2/1
  PAO2/1 -> O2 Cardiovascular Mixing and Convection Effects/2(PAO2)

== system PNEUMA/Respiratory System/Gas Exchange/DEAD SPACE ==
  PACO2 : Inport
  PAO2 : Inport  Port=2
  Flow : Inport  Port=3
  CO2 DEAD SPACE : Subsystem
  O2 DEAD SPACE : Subsystem
  Pd5CO2 : Outport
  Pd5O2 : Outport  Port=2
  wires:
  PACO2/1 -> CO2 DEAD SPACE/1(PACO2)
  PAO2/1 -> O2 DEAD SPACE/2(PAO2)
  CO2 DEAD SPACE/1(Pd5CO2) -> Pd5CO2/1
  O2 DEAD SPACE/1(Pd5O2) -> Pd5O2/1
  Flow/1 -> CO2 DEAD SPACE/2(Flow), O2 DEAD SPACE/1(Flow)

== system PNEUMA/Respiratory System/Gas Exchange/Dissociation ==
  PACO2 : Inport
  PAO2 : Inport  Port=2
  100 : Gain  Gain=100  SaturateOnIntegerOverflow=on  OutDataTypeStr=Inherit: Same as input  ParamDataTypeStr=Inherit: Same as input
  C1*Z : Gain  Gain=C1*Z  SaturateOnIntegerOverflow=on  OutDataTypeStr=Inherit: Same as input  ParamDataTypeStr=Inherit: Same as input
  CO2 Fcn -14 blocks : Fcn  Expr="(u(1) * (1+ u(2) * beta2)/((u(2) * alpha2 +1) * K2) )^(1/a2) / ( (u(1) * (1+ u(2) * beta2)/((1+ u(2) * alpha2 ) * K2) )^(1/a2)  +1) * C2*Z"
  Mux : Mux  Inputs=2
  O2 Fcn -13 blocks : Fcn  Expr="(u(2) * (1+ u(1) * beta1)/(( 1+u(1) * alpha1 ) * K1) )^(1/a1) / ( (u(2) * (1+ u(1) * beta1)/(( 1+u(1) * alpha1 ) * K1) )^(1/a1)   +1)"
  SAO2 Saturation : Saturate  UpperLimit=5  LowerLimit=-5
  CaCO2 : Outport
  SAO2 : Outport  Port=2
  CaO2 : Outport  Port=3
  wires:
  CO2 Fcn -14 blocks/1 -> CaCO2/1
  C1*Z/1 -> CaO2/1
  O2 Fcn -13 blocks/1 -> C1*Z/1, SAO2 Saturation/1
  PACO2/1 -> Mux/1
  PAO2/1 -> Mux/2
  100/1 -> SAO2/1
  SAO2 Saturation/1 -> 100/1
  Mux/1 -> CO2 Fcn -14 blocks/1, O2 Fcn -13 blocks/1

== system PNEUMA/Respiratory System/Gas Exchange/GAS EXCHANGE IN THE LUNGS ==
  CaCO2 : Inport
  CVCO2 : Inport  Port=2
  Pd5CO2 : Inport  Port=3
  Pd5O2 : Inport  Port=4
  Flow : Inport  Port=5
  Vt - Tidal Volume : Inport  Port=6
  "Q " : Inport  Port=7
  CVO2 : Inport  Port=8
  CaO2 : Inport  Port=9
  CO2 Gas Exchange in the Lungs : Subsystem
  O2 Gas Exchange in the Lungs : Subsystem
  PACO2 : Outport
  PAO2 : Outport  Port=2
  wires:
  CO2 Gas Exchange in the Lungs/1(PACO2) -> PACO2/1
  O2 Gas Exchange in the Lungs/1(PAO2) -> PAO2/1
  CaCO2/1 -> CO2 Gas Exchange in the Lungs/1(CaCO2)
  CVCO2/1 -> CO2 Gas Exchange in the Lungs/2(CVCO2)
  Pd5CO2/1 -> CO2 Gas Exchange in the Lungs/3(Pd5CO2)
  Vt - Tidal Volume/1 -> O2 Gas Exchange in the Lungs/1(Vt - Tidal Volume), CO2 Gas Exchange in the Lungs/4(Vt - Tidal Volume)
  Flow/1 -> O2 Gas Exchange in the Lungs/2(Flow), CO2 Gas Exchange in the Lungs/5(Flow)
  "Q "/1 -> O2 Gas Exchange in the Lungs/3(Q), CO2 Gas Exchange in the Lungs/6("Q ")
  CaO2/1 -> O2 Gas Exchange in the Lungs/4(CaO2)
  CVO2/1 -> O2 Gas Exchange in the Lungs/5(CVO2)
  Pd5O2/1 -> O2 Gas Exchange in the Lungs/6(Pd5O2)

== system PNEUMA/Respiratory System/Modified Upper Airway Conductance/Upper Airway Blockage ==
  Step : Step  Time=end_time  Before=1  After=0  SampleTime=0
  Step1 : Step  Time=begin_time  SampleTime=0
  Sum : Sum  Inputs=|++  InputSameDT=on  SaturateOnIntegerOverflow=on  OutDataTypeStr=Inherit: Same as first input
  Out1 : Outport
  wires:
  Sum/1 -> Out1/1
  Step1/1 -> Sum/2
  Step/1 -> Sum/1

== system PNEUMA/Respiratory System/Respiratory_Mechanics/Pleural_Pressure1 ==
  Respiratory Flow : Inport
  Vt : Inport  Port=2
  Pmus : Inport  Port=3
  "Pao " : Inport  Port=4
  Pa : Subsystem
  Pcw : Subsystem
  Sum1 : Sum  Inputs=-++  InputSameDT=on  SaturateOnIntegerOverflow=on  OutDataTypeStr=Inherit: Same as first input
  "Pleural Pressure (Ppl) " : Outport
  wires:
  Sum1/1 -> "Pleural Pressure (Ppl) "/1
  Respiratory Flow/1 -> Pcw/2(Flow), Pa/1("Flow ")
  "Pao "/1 -> Pa/2("Pao ")
  Pcw/1("Pcw ") -> Sum1/2
  Pmus/1 -> Sum1/1
  Pa/1("Pa ") -> Sum1/3
  Vt/1 -> Pcw/1(Vt)

== system PNEUMA/Respiratory System/Respiratory_Mechanics/Respiratory Muscles Activity1 ==
  RespMus Drive : Inport
  PE : Inport  Port=2
  "cond " : Inport  Port=3
  Step Size : Inport  Port=4
  Pao : Inport  Port=5
  0.25 : Gain  Gain=0.25  SaturateOnIntegerOverflow=on  OutDataTypeStr=Inherit: Same as input  ParamDataTypeStr=Inherit: Same as input
  0.5 : Gain  Gain=0.5  SaturateOnIntegerOverflow=on  OutDataTypeStr=Inherit: Same as input  ParamDataTypeStr=Inherit: Same as input
  Memory : Memory  InitialCondition=VtIC  InheritSampleTime=on
  Mux2 : Mux  Inputs=2
  Mux4 : Mux  Inputs=2
  Po_vt : Fcn  Expr=u(1)*exp(-u(2)/(0.28*VC))
  Po_vt_1 : Fcn  Expr=u(1)*exp(-u(2)/(0.28*VC))
  Product1 : Product  Inputs=**/  InputSameDT=on  SaturateOnIntegerOverflow=on  OutDataTypeStr=Inherit: Same as first input
  Product2 : Product  InputSameDT=on  SaturateOnIntegerOverflow=on  OutDataTypeStr=Inherit: Same as first input
  Product3 : Product  InputSameDT=on  SaturateOnIntegerOverflow=on  OutDataTypeStr=Inherit: Same as first input
  Resp Muscle Reaction : Subsystem
  Sum{3..4,6,8} (4 alike) : Sum  InputSameDT=on  SaturateOnIntegerOverflow=on  OutDataTypeStr=Inherit: Same as first input
  Sum5 : Sum  Inputs=-+  InputSameDT=on  SaturateOnIntegerOverflow=on  OutDataTypeStr=Inherit: Same as first input
  Sum7 : Sum  Inputs=+-  InputSameDT=on  SaturateOnIntegerOverflow=on  OutDataTypeStr=Inherit: Same as first input
  b_vt : Fcn  Expr=(1.6*VC*(7.77-exp(-u/(0.25*VC))))/(2.56+exp(-u/(0.25*VC)))
  b_vt_temp : Fcn  Expr=(1.6*VC*(7.77-exp(-u/(0.25*VC))))/(2.56+exp(-u/(0.25*VC)))
  flow generation : Subsystem
  flow generation 1 : Subsystem
  Respiratory Flow : Outport
  Vt : Outport  Port=2
  Pmus : Outport  Port=3
  wires:
  Product3/1 -> Sum4/2
  Mux2/1 -> Po_vt_1/1
  Po_vt_1/1 -> flow generation 1/1(Po_vt_1)
  Sum5/1 -> Product1/2
  Sum6/1 -> Product1/3
  Mux4/1 -> Po_vt/1
  b_vt_temp/1 -> flow generation 1/3(b_vt_1)
  flow generation 1/1(Flow_1) -> Sum3/1  "Flow_1"
  "cond "/1 -> flow generation 1/6("Cond "), flow generation/1("Cond ")
  PE/1 -> flow generation 1/4(PE_1), flow generation/3(PE), Sum7/2
  Pao/1 -> flow generation 1/5(Pao_1), flow generation/2("Pao ")
  Memory/1 -> Sum4/1
  flow generation/1(Flow) -> 0.25/1, Sum6/1, Sum3/2, Product2/2, Respiratory Flow/1  "Flow"
  Sum8/1 -> b_vt_temp/1, flow generation 1/2(Vt_1), Mux2/2
  Sum7/1 -> Pmus/1
  RespMus Drive/1 -> Resp Muscle Reaction/1(RespMus Drive)
  Product1/1 -> Sum7/1
  0.25/1 -> Sum5/1
  Sum4/1 -> Memory/1, Sum8/2, Mux4/2, flow generation/6(Vt), Vt/1, b_vt/1  "Tidal Volume"
  0.5/1 -> Product3/1
  Sum3/1 -> Product3/2
  Product2/1 -> Sum8/1
  Resp Muscle Reaction/1(Pt_frc) -> Mux2/1, Mux4/1
  Step Size/1 -> Product2/1, 0.5/1, Resp Muscle Reaction/2(Step Size)
  b_vt/1 -> Sum5/2, Sum6/2, flow generation/5(b_vt)
  Po_vt/1 -> flow generation/4("Po_vt "), Product1/1

== system PNEUMA/Respiratory System/Sleep Mechanism/Circadian High Sine Wave ==
  Gain4 : Gain  Gain=0.97  SaturateOnIntegerOverflow=on  OutDataTypeStr=Inherit: Same as input  ParamDataTypeStr=Inherit: Same as input
  Gain5 : Gain  Gain=0.22  SaturateOnIntegerOverflow=on  OutDataTypeStr=Inherit: Same as input  ParamDataTypeStr=Inherit: Same as input
  Gain6 : Gain  Gain=0.07  SaturateOnIntegerOverflow=on  OutDataTypeStr=Inherit: Same as input  ParamDataTypeStr=Inherit: Same as input
  Gain7 : Gain  Gain=0.03  SaturateOnIntegerOverflow=on  OutDataTypeStr=Inherit: Same as input  ParamDataTypeStr=Inherit: Same as input
  Gain8 : Gain  Gain=0.01  SaturateOnIntegerOverflow=on  OutDataTypeStr=Inherit: Same as input  ParamDataTypeStr=Inherit: Same as input
  Sin(2*theta) : Sin  Amplitude=0.12  Frequency=0.00014544  Phase=3.2358  SampleTime=0
  Sin(3*theta) : Sin  Amplitude=0.12  Frequency=0.00021817  Phase=3.2358  SampleTime=0
  Sin(4*theta) : Sin  Amplitude=0.12  Frequency=0.00029089  Phase=3.2358  SampleTime=0
  Sin(5*theta) : Sin  Amplitude=0.12  Frequency=0.00036361  Phase=3.2358  SampleTime=0
  Sin(theta) : Sin  Amplitude=0.12  Frequency=7.2722e-05  Phase=3.2358  SampleTime=0
  Sum : Sum  Inputs=|+++++  InputSameDT=on  SaturateOnIntegerOverflow=on  OutDataTypeStr=Inherit: Same as first input
  Sine Wave : Outport
  wires:
  Sin(theta)/1 -> Gain4/1
  Gain4/1 -> Sum/1
  Sin(2*theta)/1 -> Gain5/1
  Gain5/1 -> Sum/2
  Sin(3*theta)/1 -> Gain6/1
  Gain6/1 -> Sum/3
  Sin(4*theta)/1 -> Gain7/1
  Gain7/1 -> Sum/4
  Sin(5*theta)/1 -> Gain8/1
  Gain8/1 -> Sum/5
  Sum/1 -> Sine Wave/1

== system PNEUMA/Respiratory System/Sleep Mechanism/If Action Subsystem ==
  In1 : Inport
  Action Port : ActionPort  ActionPortLabel=if(u1 > 0)
  Out1 : Outport
  wires:
  In1/1 -> Out1/1
